simulink model "Attitude_Tracking_Quaternion"  (R2022b)
settings: Solver=VariableStepAuto  StartTime=0.0  StopTime=10.0  RelTol=1e-3
values from neighbouring files (symbols this model uses):
  q0 = angle2quat(psi0, theta0, phi0)    [Initial_condition_Integrator.m]
settings Model: Creator=mluser  LastModifiedBy=mluser

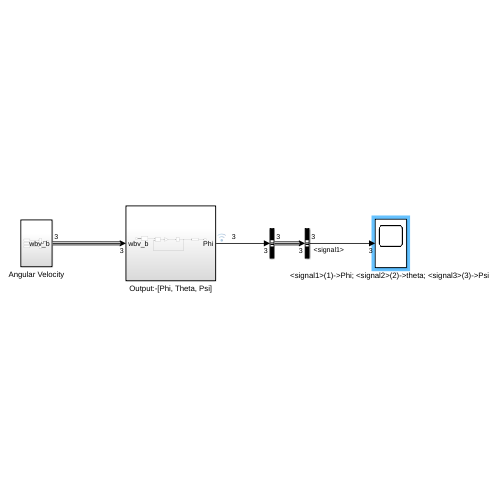
[thumbnail: Simulink's stored preview of the top-level diagram]
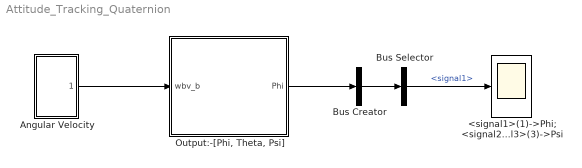
== system Attitude_Tracking_Quaternion ==
  "<signal1>(1)->Phi; <signal2>(2)->theta; <signal3>(3)->Psi " : Scope
  Angular Velocity : Subsystem
  Bus Creator : BusCreator  Inputs=1
  Bus Selector : BusSelector  OutputSignals=signal1
  "Output:-[Phi, Theta, Psi]" : Subsystem
  wires:
  Angular Velocity/1(wbv_b) -> "Output:-[Phi, Theta, Psi]"/1(wbv_b)
  Bus Creator/1 -> Bus Selector/1
  "Output:-[Phi, Theta, Psi]"/1(Phi) -> Bus Creator/1
  Bus Selector/1 -> "<signal1>(1)->Phi; <signal2>(2)->theta; <signal3>(3)->Psi "/1  "<signal1>"

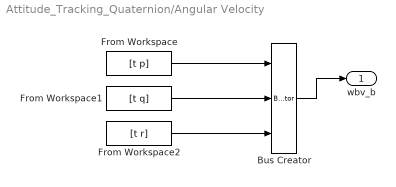
== system Attitude_Tracking_Quaternion/Angular Velocity ==
  Bus Creator : BusCreator  Inputs=3
  From Workspace : FromWorkspace  VariableName=[t p]
  From Workspace1 : FromWorkspace  VariableName=[t q]
  From Workspace2 : FromWorkspace  VariableName=[t r]
  wbv_b : Outport
  wires:
  Bus Creator/1 -> wbv_b/1
  From Workspace/1 -> Bus Creator/1
  From Workspace1/1 -> Bus Creator/2
  From Workspace2/1 -> Bus Creator/3

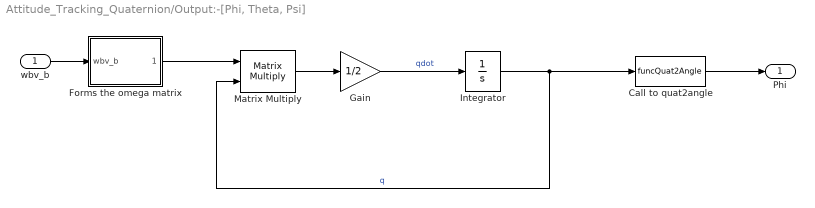
== system Attitude_Tracking_Quaternion/Output:-[Phi, Theta, Psi] ==
  wbv_b : Inport
  Call to quat2angle : MATLABFcn  MATLABFcn=funcQuat2Angle
  Forms the omega matrix : MATLAB Function  TreatAsAtomicUnit=on
  Gain : Gain  Gain=1/2
  Integrator : Integrator  InitialCondition=q0
  Matrix Multiply : Product  Multiplication=Matrix(*)
  Phi : Outport
  wires:
  wbv_b/1 -> Forms the omega matrix/1(wbv_b)
  Forms the omega matrix/1(Omega) -> Matrix Multiply/1
  Integrator/1 -> Call to quat2angle/1, Matrix Multiply/2  "q"
  Matrix Multiply/1 -> Gain/1
  Gain/1 -> Integrator/1  "qdot"
  Call to quat2angle/1 -> Phi/1

== matlab function Attitude_Tracking_Quaternion/Output:-[Phi, Theta, Psi]/Forms the omega matrix ==
  data: wbv_b input; Omega output
function Omega = fcn(wbv_b)

wx=wbv_b(1);
wy=wbv_b(2);
wz=wbv_b(3);

%Calculate Omega
Omega=[...
    0 -wx -wy -wz;
    wx 0 wz -wy;
    wy -wz 0 wx;
    wz wy -wx 0];
